simulink model "CA_3"  (Simulink 6.6)
settings: Solver=ode45  StartTime=0.0  StopTime=1e-3  RelTol=1e-3
undefined symbols (not defined in the file): get
libraries: commseqgen2 x1, dspsnks4 x1, commutil2 x1
settings Model: Creator=Мама Люда  LastModifiedBy=Мама Люда

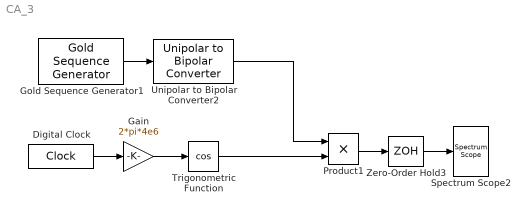
== system CA_3 ==
  Digital Clock : DigitalClock  SampleTime=5e-8
  Gain : Gain  Gain=2*pi*4e6
  Gold Sequence Generator1 : commseqgen2/Gold Sequence Generator  SystemSampleTime=-1  genPoly1=[1 0 0 1 0 0 0 0 0 0 1]  iniState1=[1 1 1 1 1 1 1 1 1 1]  genPoly2="[1 0 1 1 0  0 1 0 1 1 1]"  iniState2=[1 1 1 1 1 1 1 1 1 1]  index=0  shift=0  ts=0.9775e-6  frameBased=off  sampPerFrame=1  reset=off  outDataType=double
  Product1 : Product  RndMeth=Zero
  Spectrum Scope2 : dspsnks4/Spectrum Scope  DialogController=dspdialog.SpectrumScope  DialogControllerArgs=DataTag0  SystemSampleTime=-1  ScopeProperties=on  Domain=Frequency  HorizSpan=1  UseBuffer=on  BufferSize=1024  Overlap=0  inpFftLenInherit=off  FFTlength=128  numAvg=2  DisplayProperties=off  AxisGrid=on  Memory=off  FrameNumber=on  AxisLegend=off  AxisZoom=off  OpenScopeAtSimStart=on  OpenScopeImmediately=off  FigPos=get(0,'defaultfigureposition')  AxisProperties=off  XUnits=Hertz  XRange=[0...Fs/2]  InheritXIncr=on  XIncr=1.0  XLabel=Samples  XLimit=User-defined  YUnits=dB  XMax=6  XMin=2  YLabel=Magnitude-squared, dB  LineProperties=off  wintypeSpecScope=Bartlett  RsSpecScope=50  betaSpecScope=5  winsampSpecScope=Periodic
      settings: YMin=-34.6074307730611  YMax=10.0918649983994
  Trigonometric Function : Trigonometry  Operator=cos
  Unipolar to Bipolar Converter2 : commutil2/Unipolar to Bipolar Converter  SystemSampleTime=-1  M=2  polarity=Positive  dataType=double
  Zero-Order Hold3 : ZeroOrderHold  SampleTime=5e-8
  wires:
  Gold Sequence Generator1/1 -> Unipolar to Bipolar Converter2/1
  Unipolar to Bipolar Converter2/1 -> Product1/1
  Digital Clock/1 -> Gain/1
  Gain/1 -> Trigonometric Function/1
  Trigonometric Function/1 -> Product1/2
  Zero-Order Hold3/1 -> Spectrum Scope2/1
  Product1/1 -> Zero-Order Hold3/1
